simulink model "analisys"  (R2017b)
settings: Solver=VariableStepAuto  StartTime=0.0  StopTime=10.0  RelTol=1e-3
libraries: simulink_extras x2
settings Model: Creator=Centauro  LastModifiedBy=Centauro

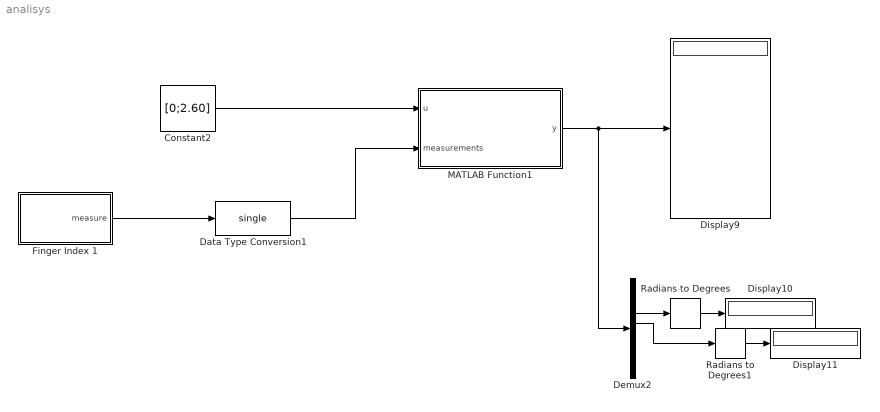
== system analisys ==
  Constant2 : Constant  Value=[0;2.60]  OutDataTypeStr=single
  Data Type Conversion1 : DataTypeConversion  OutDataTypeStr=single
  Demux2 : Demux  Outputs=8
  Display10 : Display
  Display11 : Display
  Display9 : Display
  Finger Index 1 : Subsystem
  MATLAB Function1 : MATLAB Function  TreatAsAtomicUnit=on
  Radians to Degrees : simulink_extras/Transformations/Radians to Degrees
  Radians to Degrees1 : simulink_extras/Transformations/Radians to Degrees
  wires:
  MATLAB Function1/1(y) -> Demux2/1, Display9/1
  Demux2/3 -> Radians to Degrees/1
  Demux2/4 -> Radians to Degrees1/1
  Data Type Conversion1/1 -> MATLAB Function1/2(measurements)
  Finger Index 1/1(measure) -> Data Type Conversion1/1
  Radians to Degrees/1 -> Display10/1
  Constant2/1 -> MATLAB Function1/1(u)
  Radians to Degrees1/1 -> Display11/1

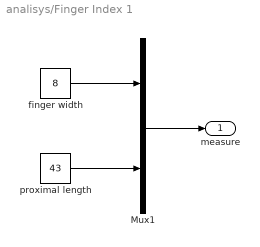
== system analisys/Finger Index 1 ==
  Mux1 : Mux  Inputs=2
  finger width : Constant  Value=8
  proximal length : Constant  Value=43
  measure : Outport
  wires:
  Mux1/1 -> measure/1
  finger width/1 -> Mux1/1
  proximal length/1 -> Mux1/2

== matlab function analisys/MATLAB Function1 ==
  data: u input; y output; measurements input
function y  = fcn(u, measurements)
%#codegen
LKNy = 19 %% MISURA
LKNx = 112 %% MISURA
LKN =  sqrt(LKNx^2 + LKNy^2); %135.6320;
qKN = atan(LKNy / LKNx); %0.1108; % angolo tra il giunto dell'attacco del motore (N) e il giunto K 


LAB =  18;
LBC =  43;
LCD =  9;
LDE =  40;
LEF =  27;
LBH =  37; 
LGH =  86;
LGF =  46;
LEJ =  39;
LCI =  16;
LKB =  35;

lact = 98; %Lunghezza dell'attuatore. [RIMISURA]
LKH = LKB + LBH;
LDF = LDE + LEF;
LBD = LBC + LCD;

xL_mag = 0; % Posizione lungo l'asse x di L rispetto a K [RIMISURA]
offset = 10; % Distanza tra il giunto K e l'appoggio del metacarpo [RIMISURA]
LIIp = measurements(1); % Semispessore del metacarpo e della falange (da tarare)
LJJp = LIIp; % semispessore della falangina (da tarare, non per forza uguale a LIIp)
LLM = measurements(2); % Lunghezza della falange

xL = -xL_mag; % Derivata  
yL = -(LIIp + offset); % Distanza tra K e 01

lx = u(1); % Allungamento del motore misurato
qB = u(2); % Angolo inB misurato dal potenziometro (espresso in radianti)

LAK = sqrt(LAB^2 + LKB^2 - 2*LAB*LKB*cos(qB)); % quadrato della distanza tra A e K. Non può venire mai negativo

%% Calcolo qK
% Calcolo di qN: l'angolo del motore (mia implementazione). Non può mai
% essere negarivo
qN = abs( acos( (- LAK^2 + LKN^2 + (lx+lact)^2)/(2*(lx+lact)*LKN) ) );

% Coseno dell'angolo in K del triangolo AKB
xK1 = (-LAB^2 + LAK^2 + LKB^2)/(2*LAK*LKB); 
qK1 = acos(xK1);

% Coseno dell'angolo in K del triangolo AKN
xK2 = (-(lx+lact)^2 + LAK^2 + LKN^2)/(2*LAK*LKN);
qK2 = acos(xK2);

% Angolo qK
qK = pi - ( qK1 + qK2 + qKN);

%% Calcolo coordinate punti cinematica parallela
% il centro del sistema di riferimento è in K con asse x verso il polso e
% asse y uscente (contratio alle dita)

% punto B
xB = - LKB * cos(qK);  yB = LKB * sin(qK);
% punto H
xH = - LKH * cos(qK);  yH = LKH * sin(qK);
% punto G
xG = xH - LGH*sin(qK);  yG = yH - LGH*cos(qK);
% punto C
xC = xB - LBC*cos(qB - qK); yC = yB - LBC * sin(qB - qK);
% punto D
xD = xC - LCD*cos(qB - qK);   yD = yC - LCD*sin(qB - qK);
% punto I
xI = xC + LCI * sin(qB - qK);   yI = yC - LCI * cos(qB - qK);
% distanza tra L ed I
LLI = sqrt((xI - xL)^2 + (yI - yL)^2);


%% C1: dello slider. Distanza I da L proiettato sullo slider
c1 = sqrt(LLI^2 - LIIp^2);

% angolo in L del triangolo LIU
xj1 = (-LIIp^2 + LLI^2 + c1^2)/(2*c1*LLI);
qj1 = abs(acos(xj1));

%% calcolo di qo1
qo1 = qj1 - atan( abs( (yL - yI)/(xL - xI) ) );
    
%% Calcolo distanze tra punti nella cinematica parallela   
LHD = sqrt((xH - xD)^2 + (yH - yD)^2);
LDG = sqrt((xG - xD)^2 + (yG - yD)^2);


% angolo in G triangolo DGH - puo' diventare ottuso
xG1 = (-LHD^2 + LDG^2 + LGH^2)/(2*LDG*LGH);
qG1 = abs(acos(xG1));
% angolo in G triangolo FGD - non puo' diventare ottuso
xG2 = (-LDF^2 + LDG^2 + LGF^2)/(2*LDG*LGF);
qG2 = abs(acos(xG2));
qG = pi - (qG1 + qG2);

%% Seconda falange
% Giunto M del dito
xM = xL - LLM*cos(qo1); yM = yL - LLM*sin(qo1);

% Angolo in D triangolo DGH
xD1 = (-LGH^2 + LHD^2 + LDG^2)/(2*LHD*LDG);
qD1 = abs(acos(xD1));
% Angolo in D triangolo GFD
xD2 = (-LGF^2 + LDG^2 + LDF^2)/(2*LDG*LDF);
qD2 = abs(acos(xD2));
% Angolo in D triangolo BDH
xD3 = (-LBH^2 + LHD^2 + LBD^2)/(2*LHD*LBD);
qD3 = abs(acos(xD3));

qD = pi - (qD1 + qD2 + qD3);

% Giunto E
xE = xD - LDE*cos(qB - qD - qK);
yE = yD - LDE*sin(qB - qD - qK);
% Giunto J
xJ = xE + LEJ*sin(qB - qD - qK);  
yJ = yE - LEJ*cos(qB - qD - qK);
% Distanza JM
LJM = sqrt((xJ - xM)^2 + (yJ - yM)^2);
% calcolo c2
c2 = sqrt(LJM^2 - LJJp^2);

% Angolo in M triangolo JSM
xj2 = (-LIIp^2 + LJM^2 + c2^2)/(2*c2*LJM);
qj2 = abs(acos(xj2));


if (xJ - xM)<=0
    qj3 = atan((yJ - yM)/(xJ - xM));
else
    qj3 = pi + atan((yJ - yM)/(xJ - xM));
end


qo2 = qj2 + qj3 - qo1;



y = [qo1; qo2; qK; qD; qG; qN; c1; c2];
